simulink model "AMR_main_model_23b"  (R2023b)
settings: Solver=FixedStepAuto  StartTime=0.0  StopTime=inf  RelTol=1e-3
model workspace (MAT data in the model file):
  RTK_health_condition = 30
  mdlWSDbList : string (value not decoded)
  min_motor_rpm = 30
  wheel_diameter = 360
undefined symbols (not defined in the file or in its folder): Down, Pull
libraries: speedgoatlib_IO60X_IO69X x12, tramontina_database_nvidialib x7, tramontina_database_curtislib x7, tramontina_database_xsenslib x4, speedgoatlib_IO691 x2, simulink x2, tramontina_database_sick_modbuslib x1, canmsglib x1
(part 2 of 2)

== system AMR_main_model_23b/CAN DB Parser Write 1/PackSubsystem ==
  In Bus Element : Inport  PortName=PackIn  Element=ID290_AMR_vehicle_speed
  AMR_vehicle_speed_lib : tramontina_database_nvidialib/CAN pack/AMR_vehicle_speed  SystemSampleTime=-1  VariantActivationTime=update diagram  AllowFlexibleInterface=on  Latency=0  AutoFrameSizeCalculation=off
  In Bus Element1 : Outport  PortName=PackOut  Element=ID290_AMR_vehicle_speed
  wires:
  In Bus Element/1 -> AMR_vehicle_speed_lib/1
  AMR_vehicle_speed_lib/1 -> In Bus Element1/1

== system AMR_main_model_23b/CAN DB Parser Write 2/BusMapping ==
  signal1 : Inport  PortName=InBus  Element=signal1
  signal2 : Inport  PortName=InBus  Element=signal2
  ID550_curtis_input_message_left.rpm_set_left : Outport  PortName=OutBus  Element=ID550_curtis_input_message_left.rpm_set_left
  ID551_curtis_input_message_right.rpm_set_right : Outport  PortName=OutBus  Element=ID551_curtis_input_message_right.rpm_set_right
  wires:
  signal1/1 -> ID550_curtis_input_message_left.rpm_set_left/1
  signal2/1 -> ID551_curtis_input_message_right.rpm_set_right/1

== system AMR_main_model_23b/CAN DB Parser Write 2/Convert2BusArray ==
  In1 : Inport  PortName=InBus  Element=ID550_curtis_input_message_left
  In2 : Inport  PortName=InBus  Element=ID551_curtis_input_message_right
  BusArray : Concatenate
  BusArrayOut : Outport
  wires:
  In1/1 -> BusArray/1
  In2/1 -> BusArray/2
  BusArray/1 -> BusArrayOut/1

== system AMR_main_model_23b/CAN DB Parser Write 2/PackSubsystem ==
  In Bus Element : Inport  PortName=PackIn  Element=ID550_curtis_input_message_left
  In Bus Element2 : Inport  PortName=PackIn  Element=ID551_curtis_input_message_right
  curtis_input_message_left_lib : tramontina_database_curtislib/CAN pack/curtis_input_message_left  SystemSampleTime=-1  VariantActivationTime=update diagram  AllowFlexibleInterface=on  Latency=0  AutoFrameSizeCalculation=off
  curtis_input_message_right_lib : tramontina_database_curtislib/CAN pack/curtis_input_message_right  SystemSampleTime=-1  VariantActivationTime=update diagram  AllowFlexibleInterface=on  Latency=0  AutoFrameSizeCalculation=off
  In Bus Element1 : Outport  PortName=PackOut  Element=ID550_curtis_input_message_left
  In Bus Element3 : Outport  PortName=PackOut  Element=ID551_curtis_input_message_right
  wires:
  In Bus Element/1 -> curtis_input_message_left_lib/1
  curtis_input_message_left_lib/1 -> In Bus Element1/1
  In Bus Element2/1 -> curtis_input_message_right_lib/1
  curtis_input_message_right_lib/1 -> In Bus Element3/1

== system AMR_main_model_23b/CAN DB Parser Write 3/Convert2BusArray ==
  In1 : Inport  PortName=InBus  Element=ID0_curtis_input_operational
  BusArray : Concatenate  NumInputs=1
  BusArrayOut : Outport
  wires:
  In1/1 -> BusArray/1
  BusArray/1 -> BusArrayOut/1

== system AMR_main_model_23b/CAN DB Parser Write 3/InputSubsystem ==
  In1_1 : Inport
  ID0_curtis_input_operational.pre_operational : Outport  PortName=OutBus  Element=ID0_curtis_input_operational.pre_operational
  wires:
  In1_1/1 -> ID0_curtis_input_operational.pre_operational/1

== system AMR_main_model_23b/CAN DB Parser Write 3/PackSubsystem ==
  In Bus Element : Inport  PortName=PackIn  Element=ID0_curtis_input_operational
  curtis_input_operational_lib : tramontina_database_curtislib/CAN pack/curtis_input_operational  SystemSampleTime=-1  VariantActivationTime=update diagram  AllowFlexibleInterface=on  Latency=0  AutoFrameSizeCalculation=off
  In Bus Element1 : Outport  PortName=PackOut  Element=ID0_curtis_input_operational
  wires:
  In Bus Element/1 -> curtis_input_operational_lib/1
  curtis_input_operational_lib/1 -> In Bus Element1/1

== system AMR_main_model_23b/CAN DB Parser Write 5/Convert2BusArray ==
  In1 : Inport  PortName=InBus  Element=ID289_mobotic_error_flag
  BusArray : Concatenate  NumInputs=1
  BusArrayOut : Outport
  wires:
  In1/1 -> BusArray/1
  BusArray/1 -> BusArrayOut/1

== system AMR_main_model_23b/CAN DB Parser Write 5/InputSubsystem ==
  In1_1 : Inport
  ID289_mobotic_error_flag.steering_unit_error : Outport  PortName=OutBus  Element=ID289_mobotic_error_flag.steering_unit_error
  wires:
  In1_1/1 -> ID289_mobotic_error_flag.steering_unit_error/1

== system AMR_main_model_23b/CAN DB Parser Write 5/PackSubsystem ==
  In Bus Element : Inport  PortName=PackIn  Element=ID289_mobotic_error_flag
  mobotic_error_flag_lib : tramontina_database_nvidialib/CAN pack/mobotic_error_flag  SystemSampleTime=-1  VariantActivationTime=update diagram  AllowFlexibleInterface=on  Latency=0  AutoFrameSizeCalculation=off
  In Bus Element1 : Outport  PortName=PackOut  Element=ID289_mobotic_error_flag
  wires:
  In Bus Element/1 -> mobotic_error_flag_lib/1
  mobotic_error_flag_lib/1 -> In Bus Element1/1

== matlab function AMR_main_model_23b/MATLAB Function1 ==
  data: Actual_Curve_Angle_Front input; Vehicle_Speed output; RPM_Speed_Left input; RPM_Speed_Right input
function Vehicle_Speed = calculateThrottleSpeed(Actual_Curve_Angle_Front, RPM_Speed_Left, RPM_Speed_Right)

    PAR_Wheel_Base = 877;
    PAR_Drive_Wheel_Offset = PAR_Wheel_Base/2;

    if Actual_Curve_Angle_Front == 0
        Vehicle_Speed = (RPM_Speed_Left + RPM_Speed_Right) / 2;
    elseif Actual_Curve_Angle_Front < 0
        Radius_C = PAR_Wheel_Base / tan(deg2rad(abs(Actual_Curve_Angle_Front)));
        Vehicle_Speed = (RPM_Speed_Left * Radius_C + RPM_Speed_Right * (Radius_C - PAR_Drive_Wheel_Offset)) / (2 * Radius_C - PAR_Drive_Wheel_Offset);
    else
        Radius_C = PAR_Wheel_Base / tan(deg2rad(abs(Actual_Curve_Angle_Front)));
        Vehicle_Speed = (RPM_Speed_Left * Radius_C + RPM_Speed_Right * (Radius_C + PAR_Drive_Wheel_Offset)) / (2 * Radius_C + PAR_Drive_Wheel_Offset);
    end
end

== stateflow chart AMR_main_model_23b/AMR_oper_mode_chart ==
  state idle
    entry:
    AMR_idle_mode = 1;
    AMR_manual_mode = 0;
    AMR_auto_mode = 0;
    exit:
    AMR_idle_mode = 0;
  state ManualMode
    entry:
    AMR_idle_mode = 0;
    AMR_manual_mode = 1;
    AMR_auto_mode = 0;
    exit:
    AMR_manual_mode = 0;
  state AutoMode
    entry:
    AMR_idle_mode = 0;
    AMR_manual_mode = 0;
    AMR_auto_mode = 1;
    exit:
    AMR_auto_mode = 0;
  (default) -> idle
  idle -> idle [order 3]
  idle -> (junction 13) [order 2] : [AMR_oper_mode == 4]
  (junction 13) -> AutoMode
  (junction 20) -> idle
  AutoMode -> (junction 20) [order 3]
  ManualMode -> idle [order 3]
  idle -> ManualMode [order 1] : [AMR_oper_mode == 2]
  ManualMode -> ManualMode [order 2] : [AMR_oper_mode == 2]
  AutoMode -> AutoMode [order 1] : [AMR_oper_mode == 4]
  ManualMode -> AutoMode [order 1] : [AMR_oper_mode == 4]
  AutoMode -> ManualMode [order 2] : [AMR_oper_mode == 2]
  data: AMR_idle_mode output; AMR_oper_mode input; AMR_manual_mode output; AMR_auto_mode output
